simulink model "DetailedModel"  (R2024b)
settings: Solver=ode23t  StartTime=0.0  StopTime=0.2  MaxStep=1e-6  RelTol=1e-4
InitFcn:
  | ModelParameters
undefined symbols (not defined in the file or in its folder): ABR, abr, dc, dc_vs, h_BTU, inv, L, setpoint, Setpoint_Harmonic_L1, time, ts, Ts_RMS
libraries: spsThreePhaseSeriesRLCBranchLib x17, spsGroundLib x14, spsControlledVoltageSourceLib x11, spsThreePhaseVIMeasurementLib x8, spsSeriesRLCBranchLib x7, eePwmGenerator x6, spsCurrentMeasurementLib x4, spsVoltageMeasurementLib x4, spsControlledCurrentSourceLib x3, eePowerMeasurement x3, spsUniversalBridgeLib x2, spsThreePhaseBreakerLib x1
(part 3 of 3)

== matlab function DetailedModel/MATLAB Function2 ==
  data: t input; a output; b output; c output
function [a, b, c] = ugrid_signal(t)
     f0 = 50.125228;
     Aa = [334.5201, 0.2502617, 1.61557, 0.1940477, 1.53563, 0.3231021, 5.360184, 0.2424031, 2.149279, 0.1007586, 0.2125878, 0.1339948, 0.5034818, 0.1263396, 0.1650067, 0.03525716, 1.135765, 0.08543849, 0.433721, 0.02282475, 0.1549782, 0.02838804,];
     Ab = [333.8043, 0.8561689, 1.797912, 0.8451434, 1.874492, 0.4650419, 5.741568, 0.4128138, 1.851249, 0.08639128, 0.3294296, 0.1806381, 0.3088068, 0.08176073, 0.6591301, 0.1429833, 1.364787, 0.1656787, 0.7980621, 0.0370358, 0.2096964, 0.07671172,];
     Ac = [332.2491, 0.06897355, 1.757924, 0.1635336, 2.219875, 0.1664537, 5.729767, 0.1672438, 1.539747, 0.1281911, 0.2675329, 0.09134745, 0.6250786, 0.0665271, 0.1723971, 0.07565897, 1.572499, 0.02511356, 0.6546616, 0.04352299, 0.2448406, 0.06000912,];
     Pa = [0.0081921, -2.1567, 1.7696, 2.0969, 2.9529, -2.2999, 0.20439, 1.5196, -3.013, -1.955, 2.7754, -0.29168, 2.2216, -2.5767, 2.999, -2.0019, 0.56989, 1.9116, 1.3808, -2.1611, 0.22434, 0.40202,];
     Pb = [-2.0842, 0.49544, 2.0406, -0.56969, -1.46, -1.9654, -1.775, -2.976, 3.0832, 0.82411, 1.5499, -0.37446, 0.4113, -2.583, -1.8131, 2.4593, 2.1101, 0.94524, -1.1132, -0.58319, 0.59708, -2.7221,];
     Pc = [2.1034, -0.85846, 1.9212, 2.9695, 1.077, -1.2956, 2.3787, -0.77043, 3.1085, -0.26472, 1.8443, 0.23393, -1.7778, 1.1371, -1.2083, 1.1489, -1.9729, 1.9068, 2.7145, 2.3886, -0.050988, 1.6189,];
     freqs = f0*[1, 2, 3, 4, 5, 6, 7, 8, 9, 10, 11, 12, 13, 14, 15, 16, 17, 18, 19, 20, 21, 22,];
     a = sum(Aa .* cos(2*pi*freqs*t + Pa));
     b = sum(Ab .* cos(2*pi*freqs*t + Pb));
     c = sum(Ac .* cos(2*pi*freqs*t + Pc));
end
%  function [a, b, c] = ugrid_signal(t)
%      f0 = 50;
%      Aa = [334.5201, 0.2502281, 1.615611, 0.1940858, 1.535643, 0.3230755, 5.360185, 0.2424435, 2.149283, 0.1007252, 0.2126131, 0.1339712, 0.5035215, 0.1263312, 0.1650277, 0.03522955, 1.135771, 0.08547964, 0.4337532, 0.02280624, 0.1549653, 0.02838129, 0.2223919, 0.07573822, 0.1624112, 0.07075177, 0.1277026, 0.03856509, 0.1036952, 0.05708784,];
%      Ab = [333.8043, 0.8561822, 1.797941, 0.8451244, 1.874461, 0.4650157, 5.74154, 0.4128148, 1.851257, 0.086408, 0.3294589, 0.1806191, 0.3088096, 0.08175423, 0.6591051, 0.14301, 1.364817, 0.1656934, 0.7980318, 0.03700917, 0.2096989, 0.07671534, 0.1886238, 0.1336484, 0.1423584, 0.06279729, 0.1335011, 0.07498264, 0.0975827, 0.05061735,];
%      Ac = [332.2489, 0.06911499, 1.757752, 0.1634846, 2.219731, 0.1666312, 5.729622, 0.1673923, 1.539699, 0.1282814, 0.2673548, 0.09136283, 0.62523, 0.06640425, 0.1725745, 0.07554177, 1.572615, 0.02493847, 0.6545196, 0.0433537, 0.2449415, 0.05985802, 0.2653508, 0.04483057, 0.07704471, 0.002056071, 0.1832673, 0.05192471, 0.119208, 0.03225567,];
%      Aa(23:26)=5;
%      Ab(23:26)=5;
%      Ac(23:26)=5;
%      Pa = [0.0081922, -2.1568, 1.7696, 2.0968, 2.9529, -2.3, 0.20439, 1.5197, -3.0131, -1.9553, 2.7752, -0.29142, 2.2216, -2.577, 2.9988, -2.0027, 0.56992, 1.9117, 1.3809, -2.1628, 0.22459, 0.40346, 1.3145, 3.061, 3.009, -0.97512, -0.19418, 1.4105, 0.077632, -2.7181,];
%      Pb = [-2.0842, 0.49547, 2.0406, -0.56966, -1.46, -1.9654, -1.775, -2.9761, 3.0832, 0.82441, 1.55, -0.37432, 0.4114, -2.5834, -1.8131, 2.4592, 2.1101, 0.9454, -1.1132, -0.5828, 0.59722, -2.7225, 2.9959, 1.2675, 0.241, 0.61834, -0.57128, -1.2753, 2.2224, 2.9746,];
%      Pc = [2.1034, -0.86005, 1.9212, 2.9706, 1.0769, -1.2957, 2.3787, -0.77102, 3.1086, -0.26592, 1.8443, 0.23199, -1.7777, 1.1352, -1.2082, 1.1472, -1.9728, 1.9058, 2.7146, 2.3897, -0.051578, 1.6174, -1.0165, 2.8124, -1.5293, -0.27296, -1.024, 3.1408, -2.1327, -0.99362,];
%      freqs = f0*[1, 2, 3, 4, 5, 6, 7, 8, 9, 10, 11, 12, 13, 14, 15, 16, 17, 18, 19, 20, 21, 22, 23, 24, 25, 26, 27, 28, 29, 30,];
%      a = sum(Aa .* cos(2*pi*freqs*t + Pa));
%      b = sum(Ab .* cos(2*pi*freqs*t + Pb));
%      c = sum(Ac .* cos(2*pi*freqs*t + Pc));
%  end
%   function [a, b, c] = ugrid_signal(t)
%      f0 = 50.0;
%      Aa = [328.284, 0.3657334, 1.992512, 0.1428231, 5.437839, 0.1118056, 4.29362, 0.07469868, 1.468165, 0.06314469, 0.2476083, 0.061553, 1.022169, 0.06313818, 0.672546, 0.02982217, 0.4055223, 0.06954966, 0.1223458, 0.02179361, 0.05048745, 0.037089, 0.08088523, 0.02172131, 0.01557499, 0.01018606, 0.2510167, 0.01302981, 0.1177864, 0.01150568,];
%      Ab = [330.0444, 0.1985026, 2.095136, 0.1727602, 4.533017, 0.1431032, 3.659779, 0.1085596, 1.990307, 0.03150273, 0.5877847, 0.02520634, 0.8129191, 0.07397922, 0.4792151, 0.07307178, 0.2033996, 0.009235279, 0.1775701, 0.04727723, 0.3652017, 0.0390289, 0.1971337, 0.01987569, 0.1465948, 0.0331587, 0.1726766, 0.01435915, 0.09774293, 0.02107418,];
%      Ac = [330.7201, 0.4352544, 2.484506, 0.212511, 4.612838, 0.07307988, 4.193284, 0.05781904, 1.690462, 0.0349032, 0.2247044, 0.03098971, 1.092426, 0.101988, 1.153638, 0.06573654, 0.6854579, 0.07706301, 0.4447445, 0.04587536, 0.2812509, 0.05660673, 0.1067389, 0.01626102, 0.03586005, 0.01650708, 0.1869377, 0.03438297, 0.08881046, 0.01595201,];
%       %    Aa(23:26)=5;
%       %Ab(23:26)=5;
%       %Ac(23:26)=5;
%      Pa = [0.033306, 2.074, 2.3079, -2.4858, -2.7802, 1.4954, 0.41555, -2.7635, -2.9559, 2.2338, -2.5448, -3.0057, 1.9185, -2.071, 2.9632, 2.3272, -0.10931, -2.9331, 1.4655, -0.69497, -1.6276, 1.5012, 1.7626, 1.3065, 2.2073, 0.24177, -0.38708, -3.0466, -0.017843, -3.0308,];
%      Pb = [-2.0572, -1.9071, 2.2885, 1.9828, -0.65524, 2.1654, -1.7753, -1.3913, -2.7601, -0.77798, -0.66519, 3.1314, 0.24124, -0.6905, 2.9962, 0.3003, 2.3522, 2.727, 1.2508, 1.9437, -1.1622, -0.92881, 0.7478, 0.25938, 1.8418, 2.1222, -0.60743, 0.84879, 1.2103, -2.3815,];
%      Pc = [2.13, -0.76973, 2.3836, 0.010315, 1.3298, 1.9757, 2.5888, 0.37828, -2.7271, 0.54834, 2.9898, 1.9377, -1.8519, 1.4367, -2.4141, -1.2667, -2.7231, 1.1826, -2.1596, -1.304, -2.8912, 2.8387, -2.8413, 1.0094, -3.0949, -0.98424, -0.73325, 2.6164, -1.9212, 0.83177,];
%      freqs = f0*[1, 2, 3, 4, 5, 6, 7, 8, 9, 10, 11, 12, 13, 14, 15, 16, 17, 18, 19, 20, 21, 22, 23, 24, 25, 26, 27, 28, 29, 30,];
%      a = sum(Aa .* cos(2*pi*freqs*t + Pa));
%      b = sum(Ab .* cos(2*pi*freqs*t + Pb));
%      c = sum(Ac .* cos(2*pi*freqs*t + Pc));
%   end
%   function [a, b, c] = ugrid_signal(t)
%      f0 = 50.0;
%      Aa = [328.284, 0.3657334, 1.992512, 0.1428231, 5.437839, 0.1118056, 4.29362, 0.07469868, 1.468165, 0.06314469, 0.2476083, 0.061553, 1.022169, 0.06313818, 0.672546, 0.02982217, 0.4055223, 0.06954966, 0.1223458, 0.02179361, 0.05048745, 0.037089, 0.08088523, 0.02172131, 0.01557499, 0.01018606, 0.2510167, 0.01302981, 0.1177864, 0.01150568,];
%      Ab = [330.0444, 0.1985026, 2.095136, 0.1727602, 4.533017, 0.1431032, 3.659779, 0.1085596, 1.990307, 0.03150273, 0.5877847, 0.02520634, 0.8129191, 0.07397922, 0.4792151, 0.07307178, 0.2033996, 0.009235279, 0.1775701, 0.04727723, 0.3652017, 0.0390289, 0.1971337, 0.01987569, 0.1465948, 0.0331587, 0.1726766, 0.01435915, 0.09774293, 0.02107418,];
%      Ac = [330.7201, 0.4352544, 2.484506, 0.212511, 4.612838, 0.07307988, 4.193284, 0.05781904, 1.690462, 0.0349032, 0.2247044, 0.03098971, 1.092426, 0.101988, 1.153638, 0.06573654, 0.6854579, 0.07706301, 0.4447445, 0.04587536, 0.2812509, 0.05660673, 0.1067389, 0.01626102, 0.03586005, 0.01650708, 0.1869377, 0.03438297, 0.08881046, 0.01595201,];
%       %Aa(4:end)=0;
%      %Ab(4:end)=0;
%      %Ac(4:end)=0;
%      Pa = [0.033306, 2.074, 2.3079, -2.4858, -2.7802, 1.4954, 0.41555, -2.7635, -2.9559, 2.2338, -2.5448, -3.0057, 1.9185, -2.071, 2.9632, 2.3272, -0.10931, -2.9331, 1.4655, -0.69497, -1.6276, 1.5012, 1.7626, 1.3065, 2.2073, 0.24177, -0.38708, -3.0466, -0.017843, -3.0308,];
%      Pb = [-2.0572, -1.9071, 2.2885, 1.9828, -0.65524, 2.1654, -1.7753, -1.3913, -2.7601, -0.77798, -0.66519, 3.1314, 0.24124, -0.6905, 2.9962, 0.3003, 2.3522, 2.727, 1.2508, 1.9437, -1.1622, -0.92881, 0.7478, 0.25938, 1.8418, 2.1222, -0.60743, 0.84879, 1.2103, -2.3815,];
%      Pc = [2.13, -0.76973, 2.3836, 0.010315, 1.3298, 1.9757, 2.5888, 0.37828, -2.7271, 0.54834, 2.9898, 1.9377, -1.8519, 1.4367, -2.4141, -1.2667, -2.7231, 1.1826, -2.1596, -1.304, -2.8912, 2.8387, -2.8413, 1.0094, -3.0949, -0.98424, -0.73325, 2.6164, -1.9212, 0.83177,];
%      freqs = f0*[1, 2, 3, 4, 5, 6, 7, 8, 9, 10, 11, 12, 13, 14, 15, 16, 17, 18, 19, 20, 21, 22, 23, 24, 25, 26, 27, 28, 29, 30,];
%      a = sum(Aa .* cos(2*pi*freqs*t + Pa));
%      b = sum(Ab .* cos(2*pi*freqs*t + Pb));
%      c = sum(Ac .* cos(2*pi*freqs*t + Pc));
%  end

== matlab function DetailedModel/MATLAB Function1 ==
  data: t input; a output; b output; c output
function [a, b, c] = ugrid_signal(t)
     f0 = 50.125228;
     Aa = [334.5201, 0.2502617, 1.61557, 0.1940477, 1.53563, 0.3231021, 5.360184, 0.2424031, 2.149279, 0.1007586, 0.2125878, 0.1339948, 0.5034818, 0.1263396, 0.1650067, 0.03525716, 1.135765, 0.08543849, 0.433721, 0.02282475, 0.1549782, 0.02838804,];
     Ab = [333.8043, 0.8561689, 1.797912, 0.8451434, 1.874492, 0.4650419, 5.741568, 0.4128138, 1.851249, 0.08639128, 0.3294296, 0.1806381, 0.3088068, 0.08176073, 0.6591301, 0.1429833, 1.364787, 0.1656787, 0.7980621, 0.0370358, 0.2096964, 0.07671172,];
     Ac = [332.2491, 0.06897355, 1.757924, 0.1635336, 2.219875, 0.1664537, 5.729767, 0.1672438, 1.539747, 0.1281911, 0.2675329, 0.09134745, 0.6250786, 0.0665271, 0.1723971, 0.07565897, 1.572499, 0.02511356, 0.6546616, 0.04352299, 0.2448406, 0.06000912,];
     Pa = [0.0081921, -2.1567, 1.7696, 2.0969, 2.9529, -2.2999, 0.20439, 1.5196, -3.013, -1.955, 2.7754, -0.29168, 2.2216, -2.5767, 2.999, -2.0019, 0.56989, 1.9116, 1.3808, -2.1611, 0.22434, 0.40202,];
     Pb = [-2.0842, 0.49544, 2.0406, -0.56969, -1.46, -1.9654, -1.775, -2.976, 3.0832, 0.82411, 1.5499, -0.37446, 0.4113, -2.583, -1.8131, 2.4593, 2.1101, 0.94524, -1.1132, -0.58319, 0.59708, -2.7221,];
     Pc = [2.1034, -0.85846, 1.9212, 2.9695, 1.077, -1.2956, 2.3787, -0.77043, 3.1085, -0.26472, 1.8443, 0.23393, -1.7778, 1.1371, -1.2083, 1.1489, -1.9729, 1.9068, 2.7145, 2.3886, -0.050988, 1.6189,];
     freqs = f0*[1, 2, 3, 4, 5, 6, 7, 8, 9, 10, 11, 12, 13, 14, 15, 16, 17, 18, 19, 20, 21, 22,];
     a = sum(Aa .* sin(2*pi*freqs*t + Pa));
     b = sum(Ab .* sin(2*pi*freqs*t + Pb));
     c = sum(Ac .* sin(2*pi*freqs*t + Pc));
end
%  function [a, b, c] = ugrid_signal(t)
%      f0 = 50;
%      Aa = [334.5201, 0.2502281, 1.615611, 0.1940858, 1.535643, 0.3230755, 5.360185, 0.2424435, 2.149283, 0.1007252, 0.2126131, 0.1339712, 0.5035215, 0.1263312, 0.1650277, 0.03522955, 1.135771, 0.08547964, 0.4337532, 0.02280624, 0.1549653, 0.02838129, 0.2223919, 0.07573822, 0.1624112, 0.07075177, 0.1277026, 0.03856509, 0.1036952, 0.05708784,];
%      Ab = [333.8043, 0.8561822, 1.797941, 0.8451244, 1.874461, 0.4650157, 5.74154, 0.4128148, 1.851257, 0.086408, 0.3294589, 0.1806191, 0.3088096, 0.08175423, 0.6591051, 0.14301, 1.364817, 0.1656934, 0.7980318, 0.03700917, 0.2096989, 0.07671534, 0.1886238, 0.1336484, 0.1423584, 0.06279729, 0.1335011, 0.07498264, 0.0975827, 0.05061735,];
%      Ac = [332.2489, 0.06911499, 1.757752, 0.1634846, 2.219731, 0.1666312, 5.729622, 0.1673923, 1.539699, 0.1282814, 0.2673548, 0.09136283, 0.62523, 0.06640425, 0.1725745, 0.07554177, 1.572615, 0.02493847, 0.6545196, 0.0433537, 0.2449415, 0.05985802, 0.2653508, 0.04483057, 0.07704471, 0.002056071, 0.1832673, 0.05192471, 0.119208, 0.03225567,];
%      Aa(23:26)=5;
%      Ab(23:26)=5;
%      Ac(23:26)=5;
%      Pa = [0.0081922, -2.1568, 1.7696, 2.0968, 2.9529, -2.3, 0.20439, 1.5197, -3.0131, -1.9553, 2.7752, -0.29142, 2.2216, -2.577, 2.9988, -2.0027, 0.56992, 1.9117, 1.3809, -2.1628, 0.22459, 0.40346, 1.3145, 3.061, 3.009, -0.97512, -0.19418, 1.4105, 0.077632, -2.7181,];
%      Pb = [-2.0842, 0.49547, 2.0406, -0.56966, -1.46, -1.9654, -1.775, -2.9761, 3.0832, 0.82441, 1.55, -0.37432, 0.4114, -2.5834, -1.8131, 2.4592, 2.1101, 0.9454, -1.1132, -0.5828, 0.59722, -2.7225, 2.9959, 1.2675, 0.241, 0.61834, -0.57128, -1.2753, 2.2224, 2.9746,];
%      Pc = [2.1034, -0.86005, 1.9212, 2.9706, 1.0769, -1.2957, 2.3787, -0.77102, 3.1086, -0.26592, 1.8443, 0.23199, -1.7777, 1.1352, -1.2082, 1.1472, -1.9728, 1.9058, 2.7146, 2.3897, -0.051578, 1.6174, -1.0165, 2.8124, -1.5293, -0.27296, -1.024, 3.1408, -2.1327, -0.99362,];
%      freqs = f0*[1, 2, 3, 4, 5, 6, 7, 8, 9, 10, 11, 12, 13, 14, 15, 16, 17, 18, 19, 20, 21, 22, 23, 24, 25, 26, 27, 28, 29, 30,];
%      a = sum(Aa .* sin(2*pi*freqs*t + Pa));
%      b = sum(Ab .* sin(2*pi*freqs*t + Pb));
%      c = sum(Ac .* sin(2*pi*freqs*t + Pc));
%  end
%   function [a, b, c] = ugrid_signal(t)
%      f0 = 50.0;
%      Aa = [328.284, 0.3657334, 1.992512, 0.1428231, 5.437839, 0.1118056, 4.29362, 0.07469868, 1.468165, 0.06314469, 0.2476083, 0.061553, 1.022169, 0.06313818, 0.672546, 0.02982217, 0.4055223, 0.06954966, 0.1223458, 0.02179361, 0.05048745, 0.037089, 0.08088523, 0.02172131, 0.01557499, 0.01018606, 0.2510167, 0.01302981, 0.1177864, 0.01150568,];
%      Ab = [330.0444, 0.1985026, 2.095136, 0.1727602, 4.533017, 0.1431032, 3.659779, 0.1085596, 1.990307, 0.03150273, 0.5877847, 0.02520634, 0.8129191, 0.07397922, 0.4792151, 0.07307178, 0.2033996, 0.009235279, 0.1775701, 0.04727723, 0.3652017, 0.0390289, 0.1971337, 0.01987569, 0.1465948, 0.0331587, 0.1726766, 0.01435915, 0.09774293, 0.02107418,];
%      Ac = [330.7201, 0.4352544, 2.484506, 0.212511, 4.612838, 0.07307988, 4.193284, 0.05781904, 1.690462, 0.0349032, 0.2247044, 0.03098971, 1.092426, 0.101988, 1.153638, 0.06573654, 0.6854579, 0.07706301, 0.4447445, 0.04587536, 0.2812509, 0.05660673, 0.1067389, 0.01626102, 0.03586005, 0.01650708, 0.1869377, 0.03438297, 0.08881046, 0.01595201,];
%       %Aa(17:26)=0;
%       %Ab(17:26)=0;
%       %Ac(17:26)=0;
%      Pa = [0.033306, 2.074, 2.3079, -2.4858, -2.7802, 1.4954, 0.41555, -2.7635, -2.9559, 2.2338, -2.5448, -3.0057, 1.9185, -2.071, 2.9632, 2.3272, -0.10931, -2.9331, 1.4655, -0.69497, -1.6276, 1.5012, 1.7626, 1.3065, 2.2073, 0.24177, -0.38708, -3.0466, -0.017843, -3.0308,];
%      Pb = [-2.0572, -1.9071, 2.2885, 1.9828, -0.65524, 2.1654, -1.7753, -1.3913, -2.7601, -0.77798, -0.66519, 3.1314, 0.24124, -0.6905, 2.9962, 0.3003, 2.3522, 2.727, 1.2508, 1.9437, -1.1622, -0.92881, 0.7478, 0.25938, 1.8418, 2.1222, -0.60743, 0.84879, 1.2103, -2.3815,];
%      Pc = [2.13, -0.76973, 2.3836, 0.010315, 1.3298, 1.9757, 2.5888, 0.37828, -2.7271, 0.54834, 2.9898, 1.9377, -1.8519, 1.4367, -2.4141, -1.2667, -2.7231, 1.1826, -2.1596, -1.304, -2.8912, 2.8387, -2.8413, 1.0094, -3.0949, -0.98424, -0.73325, 2.6164, -1.9212, 0.83177,];
%      freqs = f0*[1, 2, 3, 4, 5, 6, 7, 8, 9, 10, 11, 12, 13, 14, 15, 16, 17, 18, 19, 20, 21, 22, 23, 24, 25, 26, 27, 28, 29, 30,];
%      a = sum(Aa .* sin(2*pi*freqs*t + Pa));
%      b = sum(Ab .* sin(2*pi*freqs*t + Pb));
%      c = sum(Ac .* sin(2*pi*freqs*t + Pc));
%  end
